simulink model "Realimentacion"  (R2019a)
settings: Solver=VariableStepAuto  StartTime=0.0  StopTime=1  RelTol=1e-3
values from neighbouring files (symbols this model uses):
  k_f = acker(A,B, autov_ee)    [Berard_Modelo_ControlEE.m]
  xo = [0;0;0.5]    [Berard_Modelo_ControlEE.m]
settings Model: Creator=agusd  LastModifiedBy=ARLUBER1
settings DataIOCC: ReturnWorkspaceOutputs=off
settings DebuggingCC: ArithmeticOperatorsInVariantConditions=warning
settings SFSimCC: SimUseLocalCustomCode=off
settings RTWCC: RTWUseLocalCustomCode=off
settings CodeAppCC: StateflowObjectComments=on

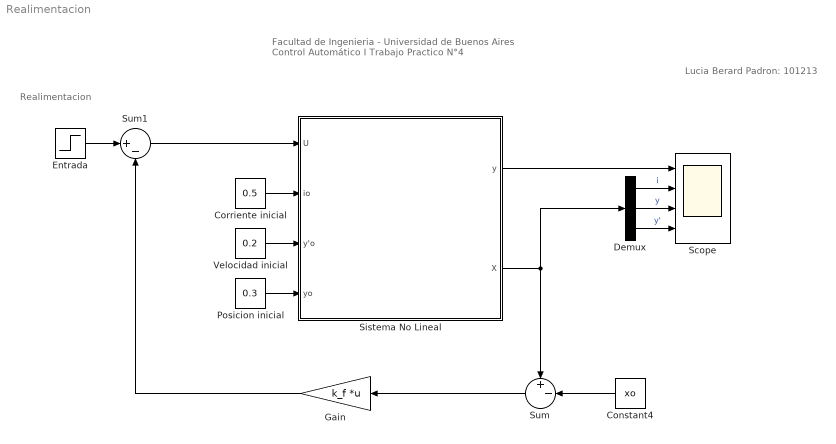
== system Realimentacion ==
  note: Lucia Berard
      | Padron: 101213
  note: Realimentacion
  note: Facultad de Ingenieria - Universidad de Buenos Aires
      | Control Automático I
      | Trabajo Practico N°4
  Constant4 : Constant  Value=xo
  Corriente inicial : Constant  Value=0.5
  Demux : Demux  Outputs=3
  Entrada : Step  Time=0  SampleTime=0.001
  Gain : Gain  Gain=k_f  Multiplication=Matrix(K*u)
  Posicion inicial : Constant  Value=0.3
  "Scope " : Scope  NumInputPorts=4
  Sistema No Lineal : Subsystem
  Sum : Sum  Inputs=+-|
  Sum1 : Sum  Inputs=|+-
  Velocidad inicial : Constant  Value=0.2
  wires:
  Corriente inicial/1 -> Sistema No Lineal/2(io)
  Velocidad inicial/1 -> Sistema No Lineal/3(y'o)
  Posicion inicial/1 -> Sistema No Lineal/4(yo)
  Demux/1 -> "Scope "/2  "i"
  Demux/2 -> "Scope "/3  "y"
  Demux/3 -> "Scope "/4  "y'"
  Sistema No Lineal/2(X) -> Demux/1, Sum/1
  Constant4/1 -> Sum/2
  Sum/1 -> Gain/1
  Gain/1 -> Sum1/2
  Sum1/1 -> Sistema No Lineal/1(U)
  Entrada/1 -> Sum1/1
  Sistema No Lineal/1("y ") -> "Scope "/1

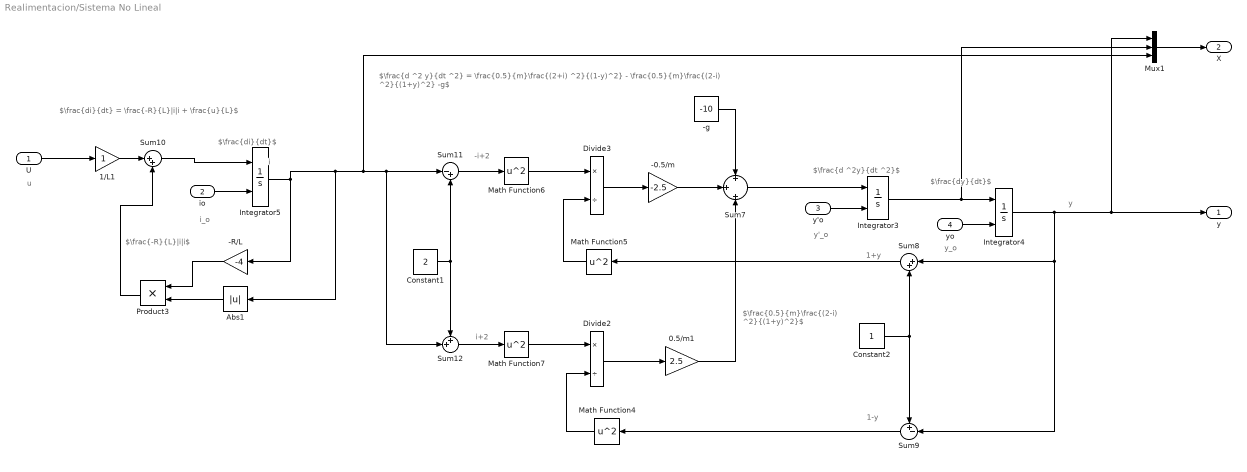
== system Realimentacion/Sistema No Lineal ==
  note: $\frac{di}{dt} = \frac{-R}{L}|i|i + \frac{u}{L}$
  note: $\frac{d ^2 y}{dt ^2} = \frac{0.5}{m}\frac{(2+i) ^2}{(1-y)^2} - \frac{0.5}{m}\frac{(2-i) ^2}{(1+y)^2} -g$
  note: i+2
  note: 1-y
  note: -i+2
  note: y
  note: i
  note: 1+y
  note: $\frac{0.5}{m}\frac{(2-i) ^2}{(1+y)^2}$
  note: y'_o
  note: y_o
  note: $\frac{-R}{L}|i|i$
  note: i_o
  note: $\frac{d ^2y}{dt ^2}$
  note: $\frac{di}{dt}$
  note: u
  note: $\frac{dy}{dt}$
  U : Inport  OutDataTypeStr=double
  io : Inport  Port=2  OutDataTypeStr=double
  y'o : Inport  Port=3
  yo : Inport  Port=4
  -0.5/m : Gain  Gain=-2.5
  -R/L : Gain  Gain=-4
  -g : Constant  Value=-10
  0.5/m1 : Gain  Gain=2.5
  1/L1 : Gain
  Abs1 : Abs
  Constant1 : Constant  Value=2
  Constant2 : Constant
  Divide2 : Product  Inputs=*/
  Divide3 : Product  Inputs=*/
  Integrator3 : Integrator  InitialConditionSource=external
  Integrator4 : Integrator  InitialConditionSource=external  UpperSaturationLimit=1  LowerSaturationLimit=-1
  Integrator5 : Integrator  InitialConditionSource=external
  Math Function{4..7} (4 alike) : Math  Operator=square  SaturateOnIntegerOverflow=on
  Mux1 : Mux  Inputs=3
  Product3 : Product
  Sum10 : Sum  Inputs=|++
  Sum11 : Sum  Inputs=|-+
  Sum12 : Sum  Inputs=++|
  Sum7 : Sum  Inputs=+|+|+
  Sum8 : Sum  Inputs=|++
  Sum9 : Sum  Inputs=+-|
  "y " : Outport
  X : Outport  Port=2
  wires:
  -g/1 -> Sum7/1
  Constant1/1 -> Sum11/2, Sum12/1
  Sum7/1 -> Integrator3/1
  Sum10/1 -> Integrator5/1
  Math Function7/1 -> Divide2/1
  0.5/m1/1 -> Sum7/3
  yo/1 -> Integrator4/2
  -0.5/m/1 -> Sum7/2
  Divide3/1 -> -0.5/m/1
  Math Function5/1 -> Divide3/2
  Math Function4/1 -> Divide2/2
  -R/L/1 -> Product3/1
  Divide2/1 -> 0.5/m1/1
  Sum8/1 -> Math Function5/1
  Sum9/1 -> Math Function4/1
  io/1 -> Integrator5/2
  Math Function6/1 -> Divide3/1
  Integrator3/1 -> Mux1/2, Integrator4/1
  Product3/1 -> Sum10/2
  Constant2/1 -> Sum9/1, Sum8/2
  U/1 -> 1/L1/1
  1/L1/1 -> Sum10/1
  Integrator4/1 -> Mux1/1, "y "/1, Sum8/1, Sum9/2
  Mux1/1 -> X/1
  Sum12/1 -> Math Function7/1
  Integrator5/1 -> Mux1/3, Sum12/2, Sum11/1, Abs1/1, -R/L/1
  y'o/1 -> Integrator3/2
  Abs1/1 -> Product3/2
  Sum11/1 -> Math Function6/1
